simulink model "homing"  (R2021a)
settings: Solver=FixedStepAuto  StartTime=0.0  StopTime=inf  FixedStep=1e-1  RelTol=1e-3
values from neighbouring files (symbols this model uses):
  MaxVelocity = 6000    [initialize_VelocityControl.m]
  PhysicalDim = 2.10667e-3    (= 0.00210667)    [initiatlize_PositionControl.m]
libraries: aerolibanimutils x2
settings Model: Creator=manue  LastModifiedBy=manue

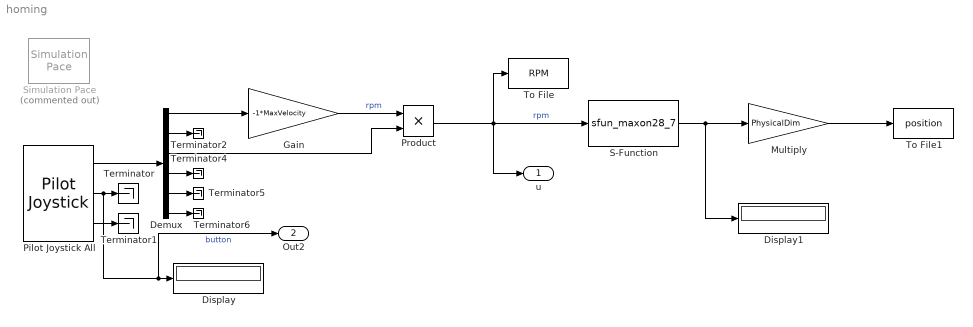
== system homing ==
  Demux : Demux  Outputs=6
  Display : Display
  Display1 : Display
  Gain : Gain  Gain=-1*MaxVelocity
  Multiply : Gain  Gain=PhysicalDim
  Pilot Joystick All : aerolibanimutils/Pilot Joystick  JoystickID=Joystick1  OutputConfiguration=AllOutputs  SampleTime=-1
  Product : Product
  S-Function : S-Function  FunctionName=sfun_maxon28_7  Parameters=NodeID, DeltaT, OperationalMode  SFunctionDeploymentMode=off  EnableBusSupport=off
  Simulation Pace : aerolibanimutils/Simulation Pace  Commented=on  SimulationPace=1  SleepMode=Auto  OutputPaceError=off  SampleTime=-1
  Terminator{,1..2,4..6} (6 alike) : Terminator
  To File : ToFile  Filename=RPM  MatrixName=rpm
  To File1 : ToFile  Filename=position  MatrixName=AbsPosition
  u : Outport
  Out2 : Outport  Port=2
  wires:
  Demux/4 -> Terminator4/1
  Pilot Joystick All/3 -> Terminator1/1
  S-Function/1 -> Display1/1, Multiply/1
  Demux/1 -> Gain/1
  Pilot Joystick All/1 -> Demux/1
  Pilot Joystick All/2 -> Out2/1, Display/1, Terminator/1  "button"
  Demux/2 -> Terminator2/1
  Demux/6 -> Terminator6/1
  Demux/5 -> Terminator5/1
  Gain/1 -> Product/1  "rpm"
  Demux/3 -> Product/2
  Product/1 -> To File/1, S-Function/1, u/1  "rpm"
  Multiply/1 -> To File1/1
